simulink model "DYN_6DOF"  (R2018b)
settings: Solver=ode3  StartTime=0.0  StopTime=50  FixedStep=0.01  RelTol=1e-3
(part 18 of 18)

== matlab function DYN_6DOF/MATLAB Function1 ==
  data: dM input; y output; C input
function y = fcn(dM,C)
x = [2,2,2,2,2,2]; % 1x6
y = x*(dM-2*C)*x';
